simulink model "px4demo_HostSerial_All_Data"  (R2016b)
settings: Solver=VariableStepAuto  StartTime=0.0  StopTime=inf  FixedStep=0.005  RelTol=1e-3  EnableMultiTasking=on
PreLoadFcn:
  | byte_size=84;
  | dt_pixhawk=1/50;
undefined symbols (not defined in the file): serial
libraries: instrumentlib x3, aerolibanimutils x1
settings Model: Creator=darenlee  LastModifiedBy=ers
settings DataIOCC: LimitDataPoints=on
settings OptimizationCC: LifeSpan=inf
settings DebuggingCC: AllowSymbolicDim=off  SFUnexpectedBacktrackingDiag=warning  SFNoUnconditionalDefaultTransitionDiag=warning  SFExecutionAtInitializationDiag=none
settings ModelReferenceCC: PropagateSignalLabelsOutOfModel=off
settings GRTTargetCC: TargetLangStandard=C89/C90 (ANSI)
settings ConfigComp: CovMetricSettings=dw  CovHtmlReporting=on  CovSaveCumulativeToWorkspaceVar=on  CovSaveSingleToWorkspaceVar=on  CovExternalEMLEnable=off

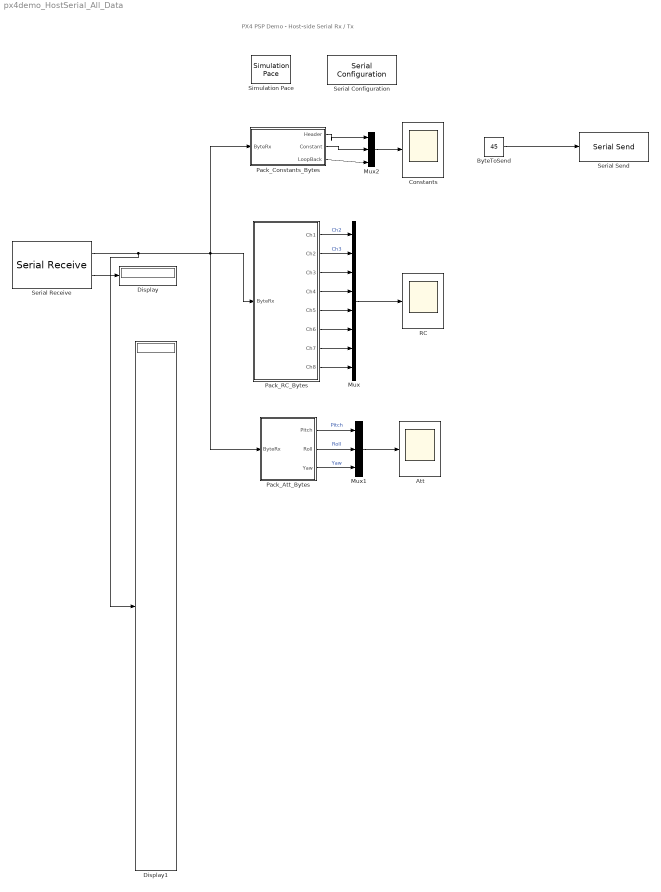
== system px4demo_HostSerial_All_Data ==
  note: PX4 PSP Demo - Host-side Serial Rx / Tx
  Att : Scope
  ByteToSend : Constant  Value=45  OutDataTypeStr=uint8  SampleTime=0.05
  Constants : Scope
  Display : Display
  Display1 : Display
      settings: Format=decimal (Stored Integer)
  Mux : Mux  Inputs=8
  Mux1 : Mux  Inputs=3
  Mux2 : Mux  Inputs=3
  Pack_Att_Bytes : Subsystem
  Pack_Constants_Bytes : Subsystem
  Pack_RC_Bytes : Subsystem
  RC : Scope
  Serial Configuration : instrumentlib/Serial Configuration  Priority=-200000  ComPortMenu=COM11  ComPort=COM11  ObjConstructor=serial('COM11');  BaudRate=115200  DataBits=8  Parity=none  StopBits=1  FlowControl=none  Timeout=10  ByteOrder=LittleEndian
  Serial Receive : instrumentlib/Serial Receive  ComPortMenu=COM11  ComPort=COM11  ObjConstructor=serial('COM11');  Terminator=<none>  DataSize="[84   1]"  DataType=uint8  EnableBlockingMode=off  ActionDataUnavailable=Output last received value  CustomValue=0  SampleTime=0.005
  Serial Send : instrumentlib/Serial Send  ComPortMenu=<Please select a port...>  ComPort=COM11  ObjConstructor=serial('COM11');  Terminator=<none>  EnableBlockingMode=off
  Simulation Pace : aerolibanimutils/Simulation Pace  SimulationPace=1  SleepMode=MATLAB Thread  OutputPaceError=off  SampleTime=0.005
  wires:
  Mux/1 -> RC/1
  Serial Receive/1 -> Display1/1, Pack_RC_Bytes/1(ByteRx), Pack_Att_Bytes/1(ByteRx), Pack_Constants_Bytes/1(ByteRx)
  Mux1/1 -> Att/1
  ByteToSend/1 -> Serial Send/1
  Serial Receive/2 -> Display/1
  Pack_Constants_Bytes/2(Constant) -> Mux2/2
  Pack_Constants_Bytes/1(Header) -> Mux2/1
  Mux2/1 -> Constants/1
  Pack_RC_Bytes/1(Ch1) -> Mux/1  "Ch2"
  Pack_RC_Bytes/4(Ch4) -> Mux/4
  Pack_RC_Bytes/5(Ch5) -> Mux/5
  Pack_RC_Bytes/6(Ch6) -> Mux/6
  Pack_RC_Bytes/7(Ch7) -> Mux/7
  Pack_RC_Bytes/2(Ch2) -> Mux/2  "Ch3"
  Pack_RC_Bytes/3(Ch3) -> Mux/3
  Pack_RC_Bytes/8(Ch8) -> Mux/8
  Pack_Att_Bytes/3(Yaw) -> Mux1/3  "Yaw"
  Pack_Att_Bytes/1(Pitch) -> Mux1/1  "Pitch"
  Pack_Att_Bytes/2(Roll) -> Mux1/2  "Roll"
  Pack_Constants_Bytes/3(LoopBack) -> Mux2/3

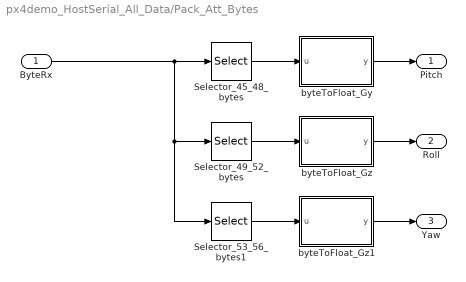
== system px4demo_HostSerial_All_Data/Pack_Att_Bytes ==
  ByteRx : Inport
  Selector_45_48_bytes : Selector  InputPortWidth=byte_size  IndexOptions=Index vector (dialog)  Indices=[45:48]  OutputSizes=1
  Selector_49_52_bytes : Selector  InputPortWidth=byte_size  IndexOptions=Index vector (dialog)  Indices=[49:52]  OutputSizes=1
  Selector_53_56_bytes1 : Selector  InputPortWidth=byte_size  IndexOptions=Index vector (dialog)  Indices=[53:56]  OutputSizes=1
  byteToFloat_Gy : MATLAB Function  TreatAsAtomicUnit=on
  byteToFloat_Gz : MATLAB Function  TreatAsAtomicUnit=on
  byteToFloat_Gz1 : MATLAB Function  TreatAsAtomicUnit=on
  Pitch : Outport
  Roll : Outport  Port=2
  Yaw : Outport  Port=3
  wires:
  byteToFloat_Gz/1(y) -> Roll/1
  ByteRx/1 -> Selector_53_56_bytes1/1, Selector_49_52_bytes/1, Selector_45_48_bytes/1
  Selector_49_52_bytes/1 -> byteToFloat_Gz/1(u)
  Selector_45_48_bytes/1 -> byteToFloat_Gy/1(u)
  byteToFloat_Gy/1(y) -> Pitch/1
  Selector_53_56_bytes1/1 -> byteToFloat_Gz1/1(u)
  byteToFloat_Gz1/1(y) -> Yaw/1

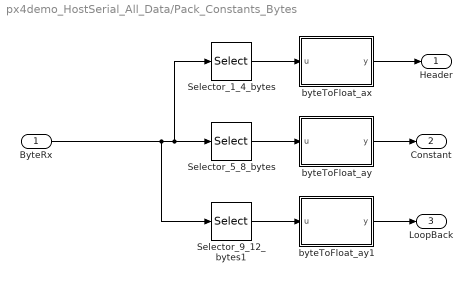
== system px4demo_HostSerial_All_Data/Pack_Constants_Bytes ==
  ByteRx : Inport
  Selector_1_4_bytes : Selector  InputPortWidth=byte_size  IndexOptions=Index vector (dialog)  Indices=[1:4]  OutputSizes=1
  Selector_5_8_bytes : Selector  InputPortWidth=byte_size  IndexOptions=Index vector (dialog)  Indices=[5 6 7 8]  OutputSizes=1
  Selector_9_12_bytes1 : Selector  InputPortWidth=byte_size  IndexOptions=Index vector (dialog)  Indices=[9 10 11 12]  OutputSizes=1
  byteToFloat_ax : MATLAB Function  TreatAsAtomicUnit=on
  byteToFloat_ay : MATLAB Function  TreatAsAtomicUnit=on
  byteToFloat_ay1 : MATLAB Function  TreatAsAtomicUnit=on
  Header : Outport
  Constant : Outport  Port=2
  LoopBack : Outport  Port=3
  wires:
  byteToFloat_ay/1(y) -> Constant/1
  Selector_5_8_bytes/1 -> byteToFloat_ay/1(u)
  Selector_1_4_bytes/1 -> byteToFloat_ax/1(u)
  byteToFloat_ax/1(y) -> Header/1
  byteToFloat_ay1/1(y) -> LoopBack/1
  Selector_9_12_bytes1/1 -> byteToFloat_ay1/1(u)
  ByteRx/1 -> Selector_9_12_bytes1/1, Selector_5_8_bytes/1, Selector_1_4_bytes/1

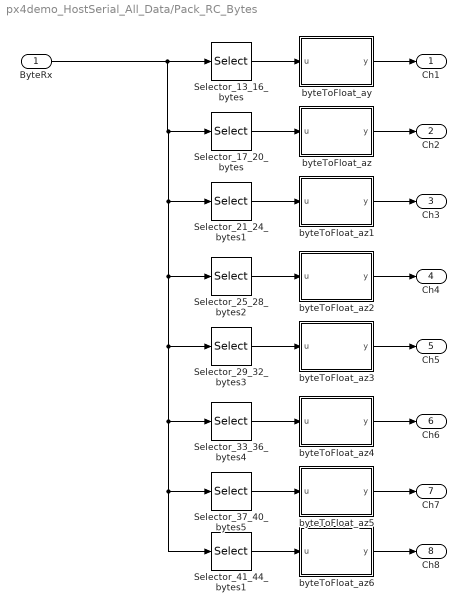
== system px4demo_HostSerial_All_Data/Pack_RC_Bytes ==
  ByteRx : Inport
  Selector_13_16_bytes : Selector  InputPortWidth=byte_size  IndexOptions=Index vector (dialog)  Indices=[13 14 15 16]  OutputSizes=1
  Selector_17_20_bytes : Selector  InputPortWidth=byte_size  IndexOptions=Index vector (dialog)  Indices=[17 18 19 20]  OutputSizes=1
  Selector_21_24_bytes1 : Selector  InputPortWidth=byte_size  IndexOptions=Index vector (dialog)  Indices=[21 22 23 24]  OutputSizes=1
  Selector_25_28_bytes2 : Selector  InputPortWidth=byte_size  IndexOptions=Index vector (dialog)  Indices=[25 26 27 28]  OutputSizes=1
  Selector_29_32_bytes3 : Selector  InputPortWidth=byte_size  IndexOptions=Index vector (dialog)  Indices=[29 30 31 32]  OutputSizes=1
  Selector_33_36_bytes4 : Selector  InputPortWidth=byte_size  IndexOptions=Index vector (dialog)  Indices=[33 34 35 36]  OutputSizes=1
  Selector_37_40_bytes5 : Selector  InputPortWidth=byte_size  IndexOptions=Index vector (dialog)  Indices=[37 38 39 40]  OutputSizes=1
  Selector_41_44_bytes1 : Selector  InputPortWidth=byte_size  IndexOptions=Index vector (dialog)  Indices=[41 42 43 44]  OutputSizes=1
  byteToFloat_ay : MATLAB Function  TreatAsAtomicUnit=on
  byteToFloat_az : MATLAB Function  TreatAsAtomicUnit=on
  byteToFloat_az1 : MATLAB Function  TreatAsAtomicUnit=on
  byteToFloat_az2 : MATLAB Function  TreatAsAtomicUnit=on
  byteToFloat_az3 : MATLAB Function  TreatAsAtomicUnit=on
  byteToFloat_az4 : MATLAB Function  TreatAsAtomicUnit=on
  byteToFloat_az5 : MATLAB Function  TreatAsAtomicUnit=on
  byteToFloat_az6 : MATLAB Function  TreatAsAtomicUnit=on
  Ch1 : Outport
  Ch2 : Outport  Port=2
  Ch3 : Outport  Port=3
  Ch4 : Outport  Port=4
  Ch5 : Outport  Port=5
  Ch6 : Outport  Port=6
  Ch7 : Outport  Port=7
  Ch8 : Outport  Port=8
  wires:
  byteToFloat_az/1(y) -> Ch2/1
  ByteRx/1 -> Selector_17_20_bytes/1, Selector_41_44_bytes1/1, Selector_37_40_bytes5/1, Selector_33_36_bytes4/1, Selector_29_32_bytes3/1, Selector_25_28_bytes2/1, Selector_21_24_bytes1/1, Selector_13_16_bytes/1
  Selector_17_20_bytes/1 -> byteToFloat_az/1(u)
  Selector_13_16_bytes/1 -> byteToFloat_ay/1(u)
  byteToFloat_ay/1(y) -> Ch1/1
  byteToFloat_az1/1(y) -> Ch3/1
  Selector_21_24_bytes1/1 -> byteToFloat_az1/1(u)
  byteToFloat_az2/1(y) -> Ch4/1
  Selector_25_28_bytes2/1 -> byteToFloat_az2/1(u)
  byteToFloat_az3/1(y) -> Ch5/1
  Selector_29_32_bytes3/1 -> byteToFloat_az3/1(u)
  byteToFloat_az4/1(y) -> Ch6/1
  Selector_33_36_bytes4/1 -> byteToFloat_az4/1(u)
  byteToFloat_az5/1(y) -> Ch7/1
  Selector_37_40_bytes5/1 -> byteToFloat_az5/1(u)
  byteToFloat_az6/1(y) -> Ch8/1
  Selector_41_44_bytes1/1 -> byteToFloat_az6/1(u)

== matlab function px4demo_HostSerial_All_Data/Pack_RC_Bytes/byteToFloat_ay ==
  data: u input; y output
function y = fcn(u)
%#codegen
y = single(0);
y = single(typecast(uint8(u),'single'));
% y = u;

== matlab function px4demo_HostSerial_All_Data/Pack_RC_Bytes/byteToFloat_az6 ==
  data: u input; y output
function y = fcn(u)
%#codegen
y = single(0);
y = single(typecast(uint8(u),'single'));
% y = u;

== matlab function px4demo_HostSerial_All_Data/Pack_RC_Bytes/byteToFloat_az ==
  data: u input; y output
function y = fcn(u)
%#codegen
y = single(0);
y = single(typecast(uint8(u),'single'));
% y = u;

== matlab function px4demo_HostSerial_All_Data/Pack_Att_Bytes/byteToFloat_Gz1 ==
  data: u input; y output
function y = fcn(u)
%#codegen
y = single(0);
y = single(typecast(uint8(u),'single'));
% y = u;

== matlab function px4demo_HostSerial_All_Data/Pack_Att_Bytes/byteToFloat_Gy ==
  data: u input; y output
function y = fcn(u)
%#codegen
y = single(0);
y = single(typecast(uint8(u),'single'));
% y = u;

== matlab function px4demo_HostSerial_All_Data/Pack_Att_Bytes/byteToFloat_Gz ==
  data: u input; y output
function y = fcn(u)
%#codegen
y = single(0);
y = single(typecast(uint8(u),'single'));
% y = u;

== matlab function px4demo_HostSerial_All_Data/Pack_Constants_Bytes/byteToFloat_ay1 ==
  data: u input; y output
function y = fcn(u)
%#codegen
y = single(0);
y = single(typecast(uint8(u),'single'));
% y = u;

== matlab function px4demo_HostSerial_All_Data/Pack_Constants_Bytes/byteToFloat_ax ==
  data: u input; y output
function y = fcn(u)
%#codegen
y = single(0);
y = single(typecast(uint8(u),'single'));
% y = u;

== matlab function px4demo_HostSerial_All_Data/Pack_Constants_Bytes/byteToFloat_ay ==
  data: u input; y output
function y = fcn(u)
%#codegen
y = single(0);
y = single(typecast(uint8(u),'single'));
% y = u;

== matlab function px4demo_HostSerial_All_Data/Pack_RC_Bytes/byteToFloat_az1 ==
  data: u input; y output
function y = fcn(u)
%#codegen
y = single(0);
y = single(typecast(uint8(u),'single'));
% y = u;

== matlab function px4demo_HostSerial_All_Data/Pack_RC_Bytes/byteToFloat_az2 ==
  data: u input; y output
function y = fcn(u)
%#codegen
y = single(0);
y = single(typecast(uint8(u),'single'));
% y = u;

== matlab function px4demo_HostSerial_All_Data/Pack_RC_Bytes/byteToFloat_az3 ==
  data: u input; y output
function y = fcn(u)
%#codegen
y = single(0);
y = single(typecast(uint8(u),'single'));
% y = u;

== matlab function px4demo_HostSerial_All_Data/Pack_RC_Bytes/byteToFloat_az4 ==
  data: u input; y output
function y = fcn(u)
%#codegen
y = single(0);
y = single(typecast(uint8(u),'single'));
% y = u;

== matlab function px4demo_HostSerial_All_Data/Pack_RC_Bytes/byteToFloat_az5 ==
  data: u input; y output
function y = fcn(u)
%#codegen
y = single(0);
y = single(typecast(uint8(u),'single'));
% y = u;
